simulink model "motorPID"  (R2019a)
settings: Solver=FixedStepAuto  StartTime=0.0  StopTime=10.0  RelTol=1e-3  EnableMultiTasking=on
undefined symbols (not defined in the file or in its folder): DiscIntNeverNeededParam
libraries: simulink x1
settings Model: Creator=florian  LastModifiedBy=florian
settings SolverCC: PositivePriorityOrder=on
settings OptimizationCC: EnhancedBackFolding=on  PassReuseOutputArgsAs=Individual arguments  MaxStackSize=64  OptimizeBlockOrder=speed  DifferentSizesBufferReuse=on  OptimizationCustomize=off
settings DebuggingCC: ParameterTunabilityLossMsg=error
settings HardwareCC: ProdBitPerPointer=32  ProdBitPerSizeT=32  ProdBitPerPtrDiffT=32  ProdLargestAtomicInteger=Long  ProdLargestAtomicFloat=Double  ProdWordSize=32  ProdLongLongMode=on  ProdHWDeviceType=ARM Compatible->ARM Cortex
settings SFSimCC: MATLABDynamicMemAlloc=off
settings RTWCC: SystemTargetFile=ert.tlc  HardwareBoard=Raspberry Pi  TLCOptions="-aInlineSetEventsForThisBaseRateFcn=TLC_FALSE -aSuppressMultiTaskScheduler=TLC_FALSE  -aRateBasedStepFcn=0"  TemplateMakefile=ert_default_tmf  GenerateReport=on  Toolchain=GNU GCC Raspberry Pi  BuildConfiguration=Faster Runs  IncludeHyperlinkInReport=on  LaunchReport=on  GenerateTraceInfo=on  GenerateTraceReport=on  GenerateTraceReportSl=on  GenerateTraceReportSf=on  GenerateTraceReportEml=on
settings CodeAppCC: ForceParamTrailComments=on  IgnoreCustomStorageClasses=off  OperatorAnnotations=on  SimulinkDataObjDesc=on  SFDataObjDesc=on  InsertBlockDesc=on
settings ERTTargetCC: SupportVariableSizeSignals=on

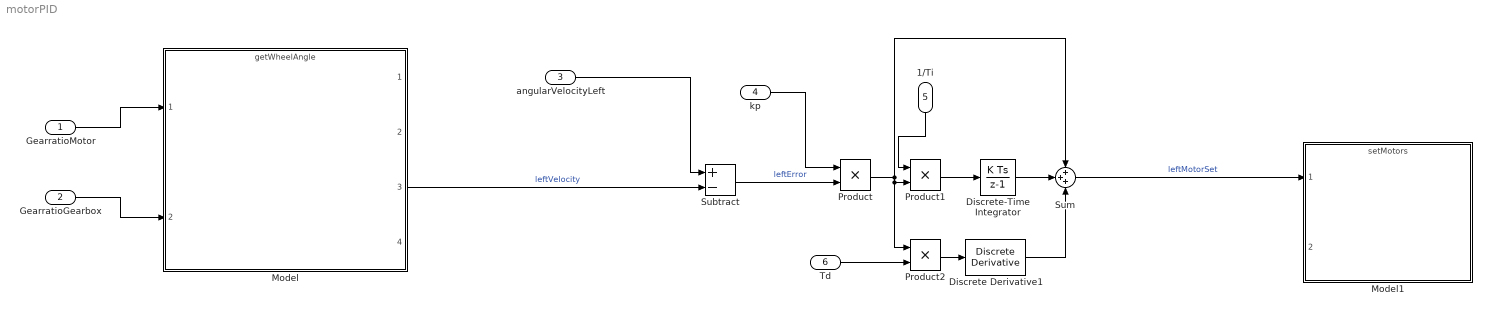
== system motorPID ==
  GearratioMotor : Inport
  GearratioGearbox : Inport  Port=2
  angularVelocityLeft : Inport  Port=3
  kp : Inport  Port=4
  1/Ti : Inport  Port=5
  Td : Inport  Port=6
  Discrete Derivative1 : simulink/Discrete/Discrete Derivative  gainval=1  ICPrevScaledInput=0.0  OutMin=[]  OutMax=[]  OutDataType=fixdt(1, 16)  OutScaling=2^-10  DoSatur=off
  Discrete-Time Integrator : DiscreteIntegrator  gainval=1  SampleTime=-1  ICPrevOutput=DiscIntNeverNeededParam  ICPrevScaledInput=DiscIntNeverNeededParam
  Model : ModelReference  ModelNameDialog=getWheelAngle.slx  SimulationMode=Normal  ModelReferenceVersion=1.42
  Model1 : ModelReference  ModelNameDialog=setMotors.slx  SimulationMode=Normal  ModelReferenceVersion=1.7
  Product : Product
  Product1 : Product
  Product2 : Product
  Subtract : Sum  Inputs=+-
  Sum : Sum  Inputs=+++
  wires:
  GearratioMotor/1 -> Model/1
  GearratioGearbox/1 -> Model/2
  angularVelocityLeft/1 -> Subtract/1
  Model/3 -> Subtract/2  "leftVelocity"
  Subtract/1 -> Product/2  "leftError"
  Product/1 -> Product2/1, Product1/2, Sum/1
  Discrete-Time Integrator/1 -> Sum/2
  Product1/1 -> Discrete-Time Integrator/1
  Discrete Derivative1/1 -> Sum/3
  Product2/1 -> Discrete Derivative1/1
  Sum/1 -> Model1/1  "leftMotorSet"
  kp/1 -> Product/1
  1/Ti/1 -> Product1/1
  Td/1 -> Product2/2
